simulink model "blu"  (Simulink 10.1)
settings: Solver=FixedStepAuto  StartTime=0.0  StopTime=100  RelTol=1e-3
values from neighbouring files (symbols this model uses):
  num = 0    [Hdb3.m]
undefined symbols (not defined in the file or in its folder): den
libraries: simulink_extras x1
settings Model: Creator=iba  LastModifiedBy=iba
settings DataIOCC: LimitDataPoints=on  DSMLogging=off  ReturnWorkspaceOutputs=on
settings OptimizationCC: DefaultParameterBehavior=Inlined  RollThreshold=2  LifeSpan=auto
settings DebuggingCC: AlgebraicLoopMsg=error  UnderspecifiedInitializationDetection=Simplified  MergeDetectMultiDrivingBlocksExec=error  SFUnexpectedBacktrackingDiag=error  SFNoUnconditionalDefaultTransitionDiag=error  SFExecutionAtInitializationDiag=warning  ArithmeticOperatorsInVariantConditions=error
settings HardwareCC: ProdBitPerPointer=64  ProdBitPerSizeT=64  ProdBitPerPtrDiffT=64  ProdLargestAtomicFloat=Float  ProdIntDivRoundTo=Zero  ProdEndianess=LittleEndian  ProdWordSize=64  ProdHWDeviceType=Intel->x86-64 (Windows64)
settings ModelReferenceCC: PropagateSignalLabelsOutOfModel=on
settings SFSimCC: SimUseLocalCustomCode=on  CustomCodeUndefinedFunction=FilterOut
settings RTWCC: RTWUseLocalCustomCode=on
settings CodeAppCC: StateflowObjectComments=off
settings GRTTargetCC: TargetLangStandard=C99 (ISO)  CombineOutputUpdateFcns=on  GRTInterface=off
settings ConfigComp: CovMetricSettings=dwe  CovHtmlReporting=off  CovSaveCumulativeToWorkspaceVar=off  CovSaveSingleToWorkspaceVar=off  CovExternalEMLEnable=on

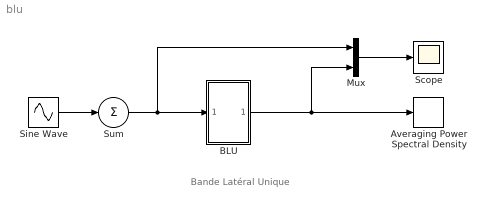
== system blu ==
  note: Bande Latéral Unique
  Averaging Power Spectral Density : simulink_extras/Additional Sinks/Averaging Power Spectral Density  npts=128*3  fftpts=512  HowOften=64  sampleT=0.1
      settings: SourceProductBaseCode=SL
  BLU : Subsystem  mask(Modulation AM){B=5, W=20}
      mask prompts: B "Fréquence Max(rad/sec)"; W "Fréquence porteuse (rad/sec)"
      mask help: Modulation d'amplitude à Bande Latérale Unique avec la méthode de Weaver
      mask init:
      | [num,den ] = butter(4,B/2,'s');
      mask Display: disp('BLU')
  Mux : Mux  Inputs=2
  Scope : Scope
  Sine Wave : Sin  Amplitude=linspace(0.15,0.1,9)  Frequency=(1:0.5:5)  SampleTime=0.1
  Sum : Sum  Inputs=+
  wires:
  Sine Wave/1 -> Sum/1
  Sum/1 -> BLU/1(In1), Mux/1
  Mux/1 -> Scope/1
  BLU/1(Out1) -> Averaging Power Spectral Density/1, Mux/2

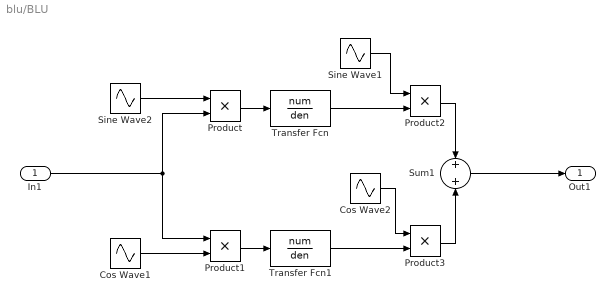
== system blu/BLU ==
  In1 : Inport
  Cos Wave1 : Sin  Frequency=B/2  Phase=pi/2  SampleTime=0
  Cos Wave2 : Sin  Frequency=W  Phase=pi/2  SampleTime=0
  Product{,1..3} (4 alike) : Product
  Sine Wave1 : Sin  Frequency=W  Samples=100  SampleTime=0
  Sine Wave2 : Sin  Frequency=B/2  Samples=100  SampleTime=0
  Sum1 : Sum
  Transfer Fcn : TransferFcn  Numerator=num  Denominator=den
  Transfer Fcn1 : TransferFcn  Numerator=num  Denominator=den
  Out1 : Outport
  wires:
  Cos Wave1/1 -> Product1/2
  Transfer Fcn1/1 -> Product3/2
  Product3/1 -> Sum1/2
  In1/1 -> Product1/1, Product/2
  Sine Wave2/1 -> Product/1
  Product1/1 -> Transfer Fcn1/1
  Cos Wave2/1 -> Product3/1
  Product2/1 -> Sum1/1
  Product/1 -> Transfer Fcn/1
  Transfer Fcn/1 -> Product2/2
  Sine Wave1/1 -> Product2/1
  Sum1/1 -> Out1/1
